simulink model "property_3_test"  (Simulink 8.4)
settings: Solver=VariableStepDiscrete  StartTime=0.0  StopTime=10.0  RelTol=1e-3
settings Model: Creator=arnaud  LastModifiedBy=arnaud
settings DataIOCC: SaveFormat=Structure
settings DebuggingCC: StrictBusMsg=Warning

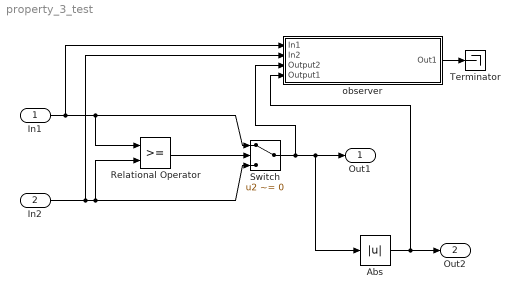
== system property_3_test ==
  In1 : Inport
  In2 : Inport  Port=2
  Abs : Abs
  Relational Operator : RelationalOperator  OutDataTypeStr=boolean
  Switch : Switch  Criteria=u2 ~= 0
  Terminator : Terminator
  observer : Subsystem  TreatAsAtomicUnit=on  mask(Observer){AnnotationType=ensures, ObserverType=ellipsoid}
      mask prompts: AnnotationType "Type of annotation (pre/post...)"; ObserverType "Observer type"
      mask help:
      | Set an observer for the system.
      | The annotation type parameter sets the type of observer:
      | - requires : pre-condition
      | - ensures : post-condition
      | - assert : an assertion
      | - observer : the observer computes a special type of properties
      mask TypeOptions AnnotationType: ensures | requires | assert | observer
      mask Callback AnnotationType:
      | paramStr = get_param(gcb, 'MaskValues');
      | 
      | if strcmp(paramStr{1}(1),'o')
      |     set_param(gcb,'MaskVisibilities',{'on';'on'});
      |     paramStr{2} = 'ellipsoid';
      |     set_param(gcb,'MaskValues',paramStr);
      | else
      |     set_param(gcb,'MaskVisibilities',{'on';'off'});
      | end
      mask Callback ObserverType:
      | paramStr = get_param(gcb, 'MaskValues');
      | 
      | if strcmp(paramStr{1}(1),'observer')
      |     set_param(gcb,'MaskVisibilities',{'on';'on'});
      |     paramStr{2} = 'ellipsoid';
      |     set_param(gcb,'MaskValues',paramStr);
      | else
      |     set_param(gcb,'MaskVisibilities',{'on';'off'});
      | end
      mask Display:
      | color('red');
      | text(0.5, 0.5, 'Observer Block', 'horizontalAlignment', 'center');
  Out1 : Outport
  Out2 : Outport  Port=2
  wires:
  In1/1 -> Relational Operator/1, Switch/1, observer/1(In1)
  In2/1 -> Relational Operator/2, Switch/3, observer/2(In2)
  Relational Operator/1 -> Switch/2
  observer/1(Out1) -> Terminator/1
  Switch/1 -> Out1/1, Abs/1, observer/3(Output2)
  Abs/1 -> Out2/1, observer/4(Output1)

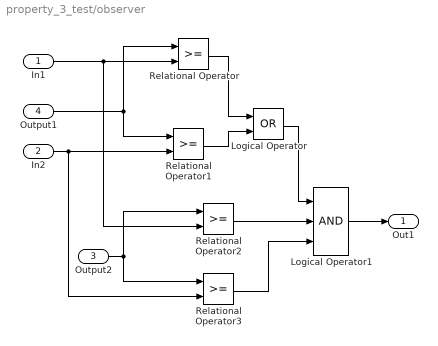
== system property_3_test/observer ==
  In1 : Inport
  In2 : Inport  Port=2
  Output2 : Inport  Port=3
  Output1 : Inport  Port=4
  Logical Operator : Logic  Operator=OR  AllPortsSameDT=off  OutDataTypeStr=boolean
  Logical Operator1 : Logic  Inputs=3  AllPortsSameDT=off  OutDataTypeStr=boolean
  Relational Operator{,1..3} (4 alike) : RelationalOperator  OutDataTypeStr=boolean
  Out1 : Outport
  wires:
  Relational Operator/1 -> Logical Operator/1
  Relational Operator1/1 -> Logical Operator/2
  Logical Operator/1 -> Logical Operator1/1
  In1/1 -> Relational Operator/2, Relational Operator2/2
  In2/1 -> Relational Operator1/2, Relational Operator3/2
  Output1/1 -> Relational Operator/1, Relational Operator1/1
  Relational Operator2/1 -> Logical Operator1/2
  Relational Operator3/1 -> Logical Operator1/3
  Output2/1 -> Relational Operator2/1, Relational Operator3/1
  Logical Operator1/1 -> Out1/1
